simulink model "HTMPC_2"  (Simulink 9.1)
settings: Solver=ode45  StartTime=0.0  StopTime=6  FixedStep=0.01  RelTol=1e-3  EnableMultiTasking=on
undefined symbols (not defined in the file): random_seeds
libraries: simulink x3, Solver_SF x1
settings Model: Creator=xuwei  LastModifiedBy=CK12
settings DataIOCC: LimitDataPoints=on
settings OptimizationCC: ExpressionDepthLimit=2147483647
settings DebuggingCC: SolverPrmCheckMsg=warning  FcnCallInpInsideContextMsg=warning  StateNameClashWarn=warning
settings ConfigComp: CovHtmlReporting=off

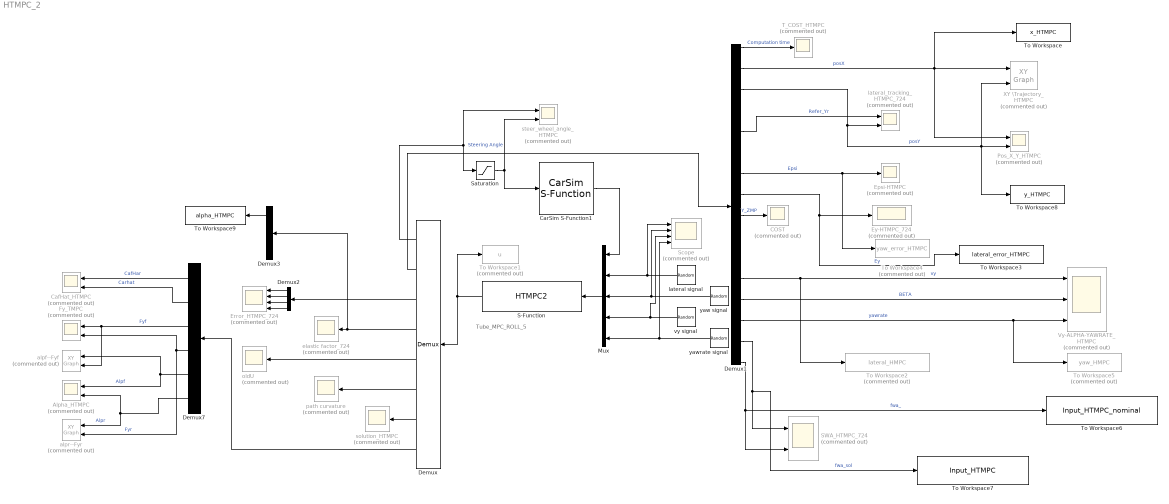
== system HTMPC_2 ==
  note: Tube_MPC_ROLL_5
  Alpha_HTMPC : Scope  Commented=on  NumInputPorts=2
  COST : Scope  Commented=on
  CafHat_HTMPC : Scope  Commented=on  NumInputPorts=2
  CarSim S-Function1 : Solver_SF/CarSim S-Function  Priority=1  SIMFILE=simfile.sim  Run_RTs=off  vs_state_ind=Run  StopMode_ind=Vehicle Model
  Demux : Demux  Outputs=[1 16 4 5 5 5 1 6]
  Demux1 : Demux  Outputs=16
  Demux2 : Demux
  Demux3 : Demux  Outputs=5
  Demux7 : Demux  Outputs=6
  Epsi-HTMPC : Scope  Commented=on
  Error_HTMPC_724 : Scope  Commented=on  NumInputPorts=4
  Ey-HTMPC_724 : Scope  Commented=on
  Fy_TMPC : Scope  Commented=on  NumInputPorts=2
  Mux : Mux  Inputs=5
  Pos_X_Y_HTMPC : Scope  Commented=on  NumInputPorts=2
  S-Function : S-Function  FunctionName=HTMPC2  SFunctionDeploymentMode=off  EnableBusSupport=off
  SWA_HTMPC_724 : Scope  Commented=on  NumInputPorts=2
  Saturation : Saturate  UpperLimit=430  LowerLimit=-430
  Scope : Scope  Commented=on  NumInputPorts=4
  T_COST_HTMPC : Scope  Commented=on
  To Workspace : ToWorkspace  VariableName=x_HTMPC  SampleTime=-1
      settings: MaxDataPoints=data_limit
  To Workspace1 : ToWorkspace  Commented=on  VariableName=u  SaveFormat=Structure  SampleTime=-1
  To Workspace2 : ToWorkspace  Commented=on  VariableName=lateral_HMPC  SaveFormat=Timeseries  SampleTime=-1
  To Workspace3 : ToWorkspace  VariableName=lateral_error_HTMPC  SampleTime=-1
      settings: MaxDataPoints=data_limit
  To Workspace4 : ToWorkspace  Commented=on  VariableName=yaw_error_HTMPC  SaveFormat=Timeseries  SampleTime=-1
  To Workspace5 : ToWorkspace  Commented=on  VariableName=yaw_HMPC  SaveFormat=Timeseries  SampleTime=-1
  To Workspace6 : ToWorkspace  VariableName=Input_HTMPC_nominal  SaveFormat=Timeseries  SampleTime=-1
  To Workspace7 : ToWorkspace  VariableName=Input_HTMPC  SampleTime=-1
      settings: MaxDataPoints=data_limit
  To Workspace8 : ToWorkspace  VariableName=y_HTMPC  SampleTime=-1
      settings: MaxDataPoints=data_limit
  To Workspace9 : ToWorkspace  VariableName=alpha_HTMPC  SampleTime=-1
      settings: MaxDataPoints=data_limit
  Vy-ALPHA-YAWRATE_HTMPC : Scope  Commented=on  NumInputPorts=3
  XY \Trajectory_HTMPC : simulink/Sinks/XY Graph  Commented=on  xmin=30  xmax=200  ymin=-0.5  ymax=4  st=-1
  alpf--Fyf : simulink/Sinks/XY Graph  Commented=on  xmin=-0.5  xmax=0.5  ymin=-10000  ymax=10000  st=-1
  alpr--Fyr : simulink/Sinks/XY Graph  Commented=on  xmin=-0.5  xmax=0.5  ymin=-8000  ymax=8000  st=-1
  elastic factor_724 : Scope  Commented=on
  lateral signal : UniformRandomNumber  Minimum=-0.05  Maximum=0.05  Seed=random_seeds  SampleTime=0.1
  lateral_tracking_HTMPC_724 : Scope  Commented=on  NumInputPorts=2
  "oldU " : Scope  Commented=on
  path curvature : Scope  Commented=on
  "solution_HTMPC " : Scope  Commented=on
  steer_wheel_angle_HTMPC : Scope  Commented=on  NumInputPorts=2
  vy signal : UniformRandomNumber  Minimum=-0.05  Maximum=0.05  Seed=random_seeds+1  SampleTime=0.1
  yaw signal : UniformRandomNumber  Minimum=-0.0174  Maximum=0.0174  Seed=random_seeds  SampleTime=0.1
  yawrate signal : UniformRandomNumber  Minimum=-0.0174  Maximum=0.0174  Seed=random_seeds+1  SampleTime=0.1
  wires:
  S-Function/1 -> To Workspace1/1, Demux/1
  Demux/1 -> steer_wheel_angle_HTMPC/1, Saturation/1
  Demux/2 -> Demux1/1
  Demux2/1 -> Error_HTMPC_724/1
  Demux2/2 -> Error_HTMPC_724/2
  Demux2/3 -> Error_HTMPC_724/3
  Demux2/4 -> Error_HTMPC_724/4
  Demux1/8 -> Ey-HTMPC_724/1, To Workspace3/1  "Ey"
  Demux1/2 -> To Workspace/1, XY \Trajectory_HTMPC/1, Pos_X_Y_HTMPC/1  "posX"
  Demux1/1 -> T_COST_HTMPC/1  "Computation time"
  Demux1/14 -> To Workspace5/1, Vy-ALPHA-YAWRATE_HTMPC/3  "yawrate"
  Demux1/3 -> XY \Trajectory_HTMPC/2, Pos_X_Y_HTMPC/2, To Workspace8/1, lateral_tracking_HTMPC_724/2  "posY"
  Demux1/7 -> To Workspace4/1, Epsi-HTMPC/1  "Epsi"
  Demux1/9 -> COST/1  "Y_ZMP"
  Demux1/12 -> Vy-ALPHA-YAWRATE_HTMPC/1, To Workspace2/1  "vy"
  Demux1/5 -> lateral_tracking_HTMPC_724/1  "Refer_Yr"
  Demux1/13 -> Vy-ALPHA-YAWRATE_HTMPC/2  "BETA"
  Demux1/15 -> SWA_HTMPC_724/1, To Workspace7/1  "fwa_sol"
  Demux1/16 -> SWA_HTMPC_724/2, To Workspace6/1  "fwa_"
  Demux/8 -> Demux7/1
  Demux7/1 -> CafHat_HTMPC/1  "CafHar"
  Demux7/2 -> CafHat_HTMPC/2  "Carhat"
  Demux7/3 -> Fy_TMPC/1, alpf--Fyf/2  "Fyf"
  Demux7/4 -> Fy_TMPC/2, alpr--Fyr/2  "Fyr"
  Demux7/5 -> alpf--Fyf/1, Alpha_HTMPC/1  "Alpf"
  Demux7/6 -> alpr--Fyr/1, Alpha_HTMPC/2  "Alpr"
  Saturation/1 -> steer_wheel_angle_HTMPC/2, CarSim S-Function1/1  "Steering Angle"
  Demux/7 -> "solution_HTMPC "/1
  Demux/6 -> path curvature/1
  Demux/4 -> Demux3/1, elastic factor_724/1
  Demux/5 -> "oldU "/1
  CarSim S-Function1/1 -> Mux/1
  Mux/1 -> S-Function/1
  lateral signal/1 -> Scope/1, Mux/2
  yaw signal/1 -> Scope/2, Mux/3
  vy signal/1 -> Scope/3, Mux/4
  yawrate signal/1 -> Scope/4, Mux/5
  Demux3/1 -> To Workspace9/1
  Demux/3 -> Demux2/1
